simulink model "pc_speaker_vc"  (R2012b)
settings: Solver=ode4  StartTime=0.0  StopTime=10.0  FixedStep=0.01  RelTol=1e-3
settings Model: SimulationMode=external  Creator=inteco  LastModifiedBy=inteco
settings RTWCC: SystemTargetFile=rtcon_tras_usb2.tlc  TemplateMakefile=rtcon_tras_vc_usb2_x64.tmf  Description=TRAS RTDAC/USB2 (Visual C/C++)  ProcessScript=rtcon_tras_usb2_make_rtw_hook
settings STFCustomTargetCC: CodeReplacementLibrary=ANSI_C  ModelReferenceCompliant=off  GeneratePreprocessorConditionals=Disable all  CombineOutputUpdateFcns=on  MatFileLogging=on  GRTInterface=off  SystemTargetFile=rtcon_tras_usb2.tlc
settings GRTTargetCC: ModelReferenceCompliant=off  ParMdlRefBuildCompliant=off  CompOptLevelCompliant=off  ConcurrentExecutionCompliant=off  ExtMode=on  ExtModeMexFile=rtcon_ext_comm

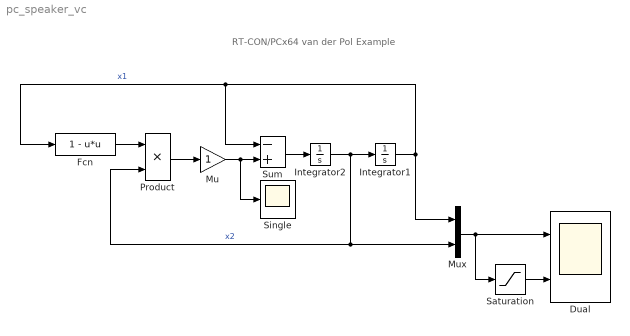
== system pc_speaker_vc ==
  note: RT-CON/PCx64 van der Pol Example
  Dual : Scope  NumInputPorts=2
      settings: TimeRange=10  YMin=-3~-5  YMax=5~5
  Fcn : Fcn  Expr=1 - u*u
  Integrator1 : Integrator  InitialCondition=2
  Integrator2 : Integrator
  Mu : Gain  SaturateOnIntegerOverflow=on  OutDataTypeStr=Inherit: Same as input  ParamDataTypeStr=Inherit: Same as input
  Mux : Mux  Inputs=2
  Product : Product  SaturateOnIntegerOverflow=on  RndMeth=Zero  InputSameDT=on  OutDataTypeStr=Inherit: Same as first input
  Saturation : Saturate  UpperLimit=2  LowerLimit=-2
  Single : Scope
      settings: TimeRange=10  YMin=-10  YMax=7.5
  Sum : Sum  Inputs=-+  SaturateOnIntegerOverflow=on  InputSameDT=on  OutDataTypeStr=Inherit: Same as first input
  wires:
  Sum/1 -> Integrator2/1
  Integrator2/1 -> Integrator1/1, Product/2, Mux/2  "x2"
  Integrator1/1 -> Mux/1, Fcn/1, Sum/1  "x1"
  Product/1 -> Mu/1
  Mu/1 -> Sum/2, Single/1
  Fcn/1 -> Product/1
  Saturation/1 -> Dual/2
  Mux/1 -> Saturation/1, Dual/1
